simulink model "OrbitPropagatorBlockExampleModel"  (R2021a)
settings: Solver=ode23t  StartTime=0.0  StopTime=21600  FixedStep=5  MinStep=10  RelTol=1e-5  AbsTol=1e-6
model workspace (MATLAB code in the model file):
  | initialize6DOFSkyHogg;
settings Model: Creator=The MathWorks, Inc.  LastModifiedBy=The MathWorks, Inc.
settings SolverCC: MaxConsecutiveMinStep=5  AlgebraicLoopSolver=TrustRegion  AutoInsertRateTranBlk=on  InsertRTBMode=Never (minimum delay)  MinimalZcImpactIntegration=on
settings DataIOCC: SignalLogging=off  DSMLogging=off  SaveTime=off
settings OptimizationCC: EnhancedBackFolding=on  StrengthReduction=on  InitFltsAndDblsToZero=on  DifferentSizesBufferReuse=on
settings DebuggingCC: WriteAfterWriteMsg=DisableAll  AlgebraicLoopMsg=none  FcnCallInpInsideContextMsg=warning  UnconnectedInputMsg=none  UnconnectedOutputMsg=none  UnconnectedLineMsg=none  UniqueDataStoreMsg=error  RootOutportRequireBusObject=none  StateNameClashWarn=warning  PregeneratedLibrarySubsystemCodeDiagnostic=none  StrictBusMsg=ErrorOnBusTreatedAsVector  SFUnexpectedBacktrackingDiag=warning  SFNoUnconditionalDefaultTransitionDiag=warning  SFExecutionAtInitializationDiag=none  SFMachineParentedDataDiag=warning  ArithmeticOperatorsInVariantConditions=warning
settings ModelReferenceCC: PropagateSignalLabelsOutOfModel=off
settings SFSimCC: SimUseLocalCustomCode=off
settings RTWCC: RTWUseLocalCustomCode=off
settings CodeAppCC: StateflowObjectComments=on

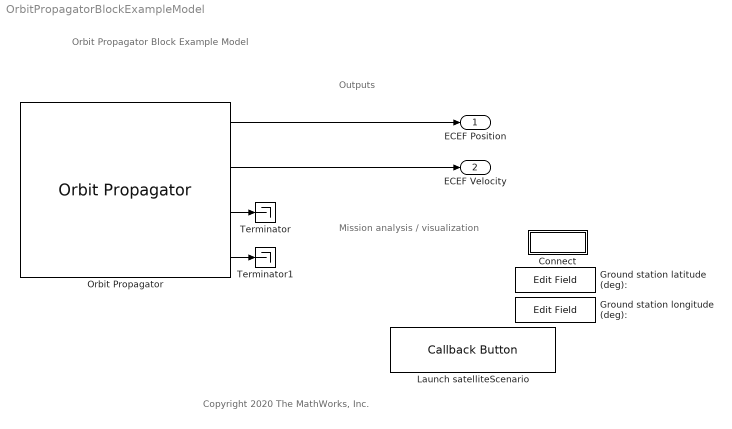
== system OrbitPropagatorBlockExampleModel ==
  note: Copyright 2020 The MathWorks, Inc.
  note: Orbit Propagator Block Example Model
  note: Mission analysis / visualization
  note: Outputs
  Connect : Subsystem
      mask Display: disp("Edit box\nconnections")
  Ground station latitude (deg): : EditField  LabelPosition=Hide  ShowInitialText=on  Alignment=Center
  Ground station longitude (deg): : EditField  LabelPosition=Hide  ShowInitialText=on  Alignment=Center
  Launch satelliteScenario : CallbackButton  ButtonText=Run model and open Satellite Scenario Viewer
      settings: ClickFcn=|
      | % Find orbit propagator block in model
      | cb.mdl = bdroot(gcb);
      | cb.blk = Simulink.findBlocksOfType(cb.mdl,"OrbitPropagator");
      | 
      | % Create Simulation input object to run model
      | cb.simInput = Simulink.SimulationInput(cb.mdl);
      | cb.simInput = setModelParameter(cb.simInput, ...
      |     "SolverType", "Variable-step", "SolverName", "VariableStepAuto", ...
      |     "RelTol", "1e-7", "AbsTol", "1e-8", ...
      |     "SaveOutput", "on", "OutputSaveName", "yout", ...
      |     "SaveFormat", "Dataset");
      | 
      | % Run the model
      | cb.out = sim(cb.simInput);
      | 
      | % Extract timeseries data from Simulation output object
      | cb.timeseriesPosECEF = cb.out.yout{1}.Values;
      | cb.timeseriesPosECEF.TimeInfo.StartDate = ...
      |     datetime(eval(get_param(cb.blk,'startDate')), "convertFrom", "juliandate");
      | cb.timeseriesVelECEF = cb.out.yout{2}.Values;
      | 
      | % Create satellite scenario
      | scenario_OrbitPropExample = satelliteScenario;
      | 
      | % Add satellites from timeseries data
      | cb.tsSize = size(cb.timeseriesPosECEF.Data);
      | cb.numSats = cb.tsSize(cb.tsSize ~= cb.timeseriesPosECEF.Length & cb.tsSize ~= 3);
      | if isempty(cb.numSats); cb.numSats = 3; end
      | cb.names = "Satellite " + (1:cb.numSats);
      | cb.sat = satellite(scenario_OrbitPropExample, cb.timeseriesPosECEF, cb.timeseriesVelECEF, ...
      |     "CoordinateFrame", "ecef", "Name", cb.names);
      | 
      | % Set satellite graphical properties
      | cb.colorMap = lines(256); cb.colorMap(1:3, :) = [];
      | for cbidx = 1:numel(cb.sat)
      |     cb.sat(cbidx).Orbit.LineColor = cb.colorMap(cbidx,:);
      |     cb.sat(cbidx).MarkerColor = cb.colorMap(cbidx,:);
      |     cb.sat(cbidx).LabelFontColor = cb.colorMap(cbidx,:);
      |     cb.sat(cbidx).GroundTrack.LeadLineColor = cb.colorMap(cbidx,:);
      | end
      | 
      | % Add ground station to scenario
      | cb.gs = groundStation(scenario_OrbitPropExample, str2double(get_param(cb.mdl+"/Connect/LatVal", "Value")),...
      |    str2double(get_param(cb.mdl+"/Connect/LonVal", "Value")), "MinElevationAngle", 10, ...
      |    "Name", "Ground Station");
      | 
      | % Add access analysis between each satellite and the ground station
      | for cbidx = 1:numel(cb.sat)
      |     cb.ac(cbidx) = access(cb.sat(cbidx), cb.gs);
      |     cb.ac(cbidx).LineColor = "green";
      | end
      | 
      | % Clean up variables created in base workspace
      | clear cb cbidx;
      | 
      | % Open and animate scenario
      | play(scenario_OrbitPropExample);
      | 
      | % Scenario object scenario_OrbitPropExample is in the base workspace for further analysis
  Orbit Propagator : OrbitPropagator  propagator=Numerical (high precision)  outportFrame=Fixed-frame  semiMajorAxis=[6786000 10000000]  eccentricity=[0.01 .2]  inclination=[50 95]  raan=[95 75]  argPeriapsis=[93 120]  trueAnomaly=[203 100]  customMu=4.305e13  customJ2=1.0826269e-03  outputTransform=on
      settings: AttributesFormatString=|
      | %<propagator>
      | Earth gravity: %<gravityModel>
      | Output coordinate system: %<outportFrame>
  Terminator : Terminator
  Terminator1 : Terminator
  ECEF Position : Outport
  ECEF Velocity : Outport  Port=2
  wires:
  Orbit Propagator/4 -> Terminator1/1
  Orbit Propagator/3 -> Terminator/1
  Orbit Propagator/1 -> ECEF Position/1
  Orbit Propagator/2 -> ECEF Velocity/1

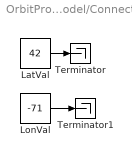
== system OrbitPropagatorBlockExampleModel/Connect ==
  LatVal : Constant  Value=42
  LonVal : Constant  Value=-71
  Terminator : Terminator
  Terminator1 : Terminator
  wires:
  LatVal/1 -> Terminator/1
  LonVal/1 -> Terminator1/1
